simulink model "PI"  (R2020a)
settings: Solver=ode4  StartTime=0.0  StopTime=5  FixedStep=1e-3  RelTol=1e-3
values from neighbouring files (symbols this model uses):
  A = w0 * [0 1 -1 ... (first row only)    [HMPC01_mult_shooting.m]
  B = [0;gamma;0]    [HMPC01_mult_shooting.m]
  C = [0 0 w0]    [HMPC01_mult_shooting.m]
  K = Kh(1:3)    [HMPC01_mult_shooting.m]
  ki = -Kh(4)    [HMPC01_mult_shooting.m]
settings Model: Creator=helon  LastModifiedBy=helon

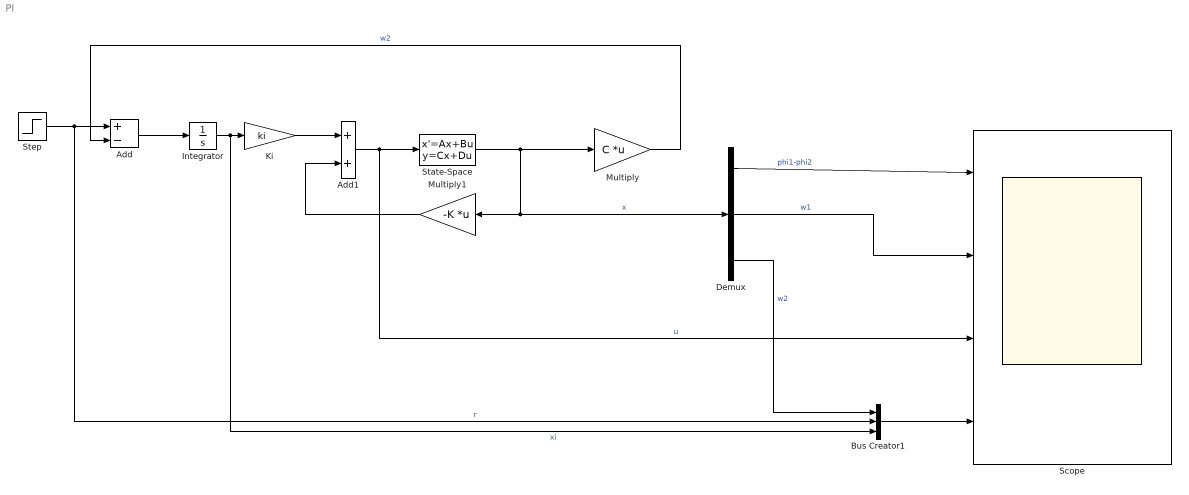
== system PI ==
  Add : Sum  Inputs=+-
  Add1 : Sum
  Bus Creator1 : BusCreator  Inputs=3
  Demux : Demux  Outputs=3
  Integrator : Integrator
  Ki : Gain  Gain=ki
  Multiply : Gain  Gain=C  Multiplication=Matrix(K*u)
  Multiply1 : Gain  Gain=-K  Multiplication=Matrix(K*u)
  Scope : Scope  NumInputPorts=4
  State-Space : StateSpace  A=A  B=B  C=eye(3)  D=zeros(3,1)  InitialCondition=0
  Step : Step  Time=0  SampleTime=0
  wires:
  State-Space/1 -> Multiply1/1, Demux/1, Multiply/1  "x"
  Step/1 -> Bus Creator1/2, Add/1  "r"
  Add/1 -> Integrator/1
  Integrator/1 -> Bus Creator1/3, Ki/1  "xi"
  Ki/1 -> Add1/1
  Add1/1 -> Scope/3, State-Space/1  "u"
  Multiply/1 -> Add/2  "w2"
  Multiply1/1 -> Add1/2
  Demux/1 -> Scope/1  "phi1-phi2"
  Demux/2 -> Scope/2  "w1"
  Demux/3 -> Bus Creator1/1  "w2"
  Bus Creator1/1 -> Scope/4
